simulink model "Charging_After_Balancing_16S1P"  (R2024b)
settings: Solver=VariableStepAuto  StartTime=0.0  StopTime=2500  RelTol=1e-3
undefined symbols (not defined in the file): Ion, Lithium
libraries: spsCurrentMeasurementLib x18, spsSeriesRLCBranchLib x17, spsVoltageMeasurementLib x17, spsBatteryLib x16, spsMosfetLib x16, spsIdealSwitchLib x2, spsDCVoltageSourceLib x1, spspowerguiLib x1
settings Model: SimulationMode=accelerator  Creator=HP
settings RTWCC: GPUComputeCapability=3.5

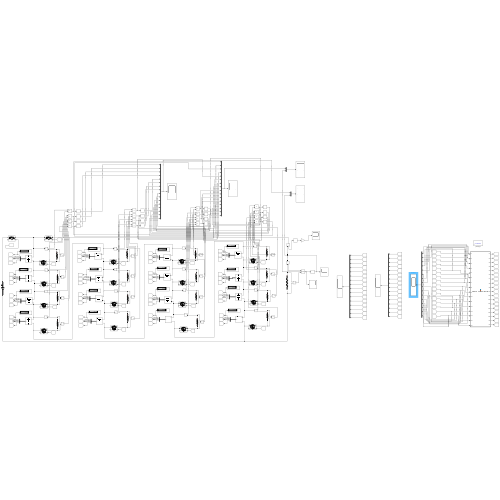
[thumbnail: Simulink's stored preview of the top-level diagram]
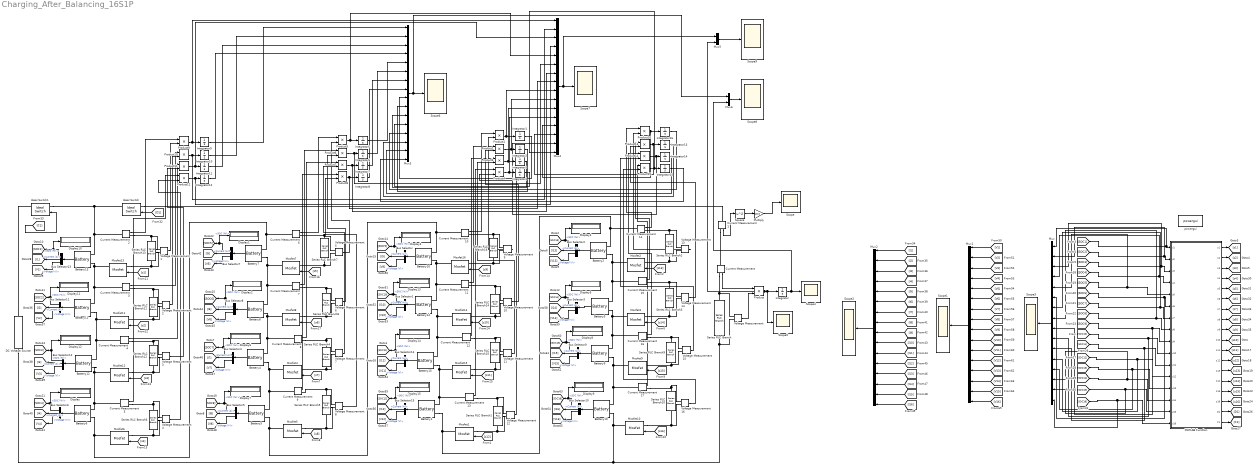
== system Charging_After_Balancing_16S1P ==
  Battery1 : spsBatteryLib/Battery  BatType=Lithium-Ion  NomV=3.3  NomQ=2.6  SOC=59  Batt_Tr=30  PresetModel=on  MaxQ=2.6  MinV=2.475  FullV=3.8412  Dis_rate=1.1304  R=0.012692  Normal_OP=2.3513  expZone="[3.5653     0.12774]"
  Battery10 : spsBatteryLib/Battery  BatType=Lithium-Ion  NomV=3.3  NomQ=2.6  SOC=55  Batt_Tr=30  PresetModel=on  MaxQ=2.6  MinV=2.475  FullV=3.8412  Dis_rate=1.1304  R=0.012692  Normal_OP=2.3513  expZone="[3.5653     0.12774]"
  Battery11 : spsBatteryLib/Battery  BatType=Lithium-Ion  NomV=3.3  NomQ=2.6  SOC=69  Batt_Tr=30  PresetModel=on  MaxQ=2.6  MinV=2.475  FullV=3.8412  Dis_rate=1.1304  R=0.012692  Normal_OP=2.3513  expZone="[3.5653     0.12774]"
  Battery12 : spsBatteryLib/Battery  BatType=Lithium-Ion  NomV=3.3  NomQ=2.6  SOC=68  Batt_Tr=30  PresetModel=on  MaxQ=2.6  MinV=2.475  FullV=3.8412  Dis_rate=1.1304  R=0.012692  Normal_OP=2.3513  expZone="[3.5653     0.12774]"
  Battery13 : spsBatteryLib/Battery  BatType=Lithium-Ion  NomV=3.3  NomQ=2.6  SOC=70  Batt_Tr=30  PresetModel=on  MaxQ=2.6  MinV=2.475  FullV=3.8412  Dis_rate=1.1304  R=0.012692  Normal_OP=2.3513  expZone="[3.5653     0.12774]"
  Battery14 : spsBatteryLib/Battery  BatType=Lithium-Ion  NomV=3.3  NomQ=2.6  SOC=61  Batt_Tr=30  PresetModel=on  MaxQ=2.6  MinV=2.475  FullV=3.8412  Dis_rate=1.1304  R=0.012692  Normal_OP=2.3513  expZone="[3.5653     0.12774]"
  Battery15 : spsBatteryLib/Battery  BatType=Lithium-Ion  NomV=3.3  NomQ=2.6  SOC=60  Batt_Tr=30  PresetModel=on  MaxQ=2.6  MinV=2.475  FullV=3.8412  Dis_rate=1.1304  R=0.012692  Normal_OP=2.3513  expZone="[3.5653     0.12774]"
  Battery16 : spsBatteryLib/Battery  BatType=Lithium-Ion  NomV=3.3  NomQ=2.6  SOC=62  Batt_Tr=30  PresetModel=on  MaxQ=2.6  MinV=2.475  FullV=3.8412  Dis_rate=1.1304  R=0.012692  Normal_OP=2.3513  expZone="[3.5653     0.12774]"
  Battery2 : spsBatteryLib/Battery  BatType=Lithium-Ion  NomV=3.3  NomQ=2.6  SOC=58  Batt_Tr=30  PresetModel=on  MaxQ=2.6  MinV=2.475  FullV=3.8412  Dis_rate=1.1304  R=0.012692  Normal_OP=2.3513  expZone="[3.5653     0.12774]"
  Battery3 : spsBatteryLib/Battery  BatType=Lithium-Ion  NomV=3.3  NomQ=2.6  SOC=57  Batt_Tr=30  PresetModel=on  MaxQ=2.6  MinV=2.475  FullV=3.8412  Dis_rate=1.1304  R=0.012692  Normal_OP=2.3513  expZone="[3.5653     0.12774]"
  Battery4 : spsBatteryLib/Battery  BatType=Lithium-Ion  NomV=3.3  NomQ=2.6  SOC=64  Batt_Tr=30  PresetModel=on  MaxQ=2.6  MinV=2.475  FullV=3.8412  Dis_rate=1.1304  R=0.012692  Normal_OP=2.3513  expZone="[3.5653     0.12774]"
  Battery5 : spsBatteryLib/Battery  BatType=Lithium-Ion  NomV=3.3  NomQ=2.6  SOC=63  Batt_Tr=30  PresetModel=on  MaxQ=2.6  MinV=2.475  FullV=3.8412  Dis_rate=1.1304  R=0.012692  Normal_OP=2.3513  expZone="[3.5653     0.12774]"
  Battery6 : spsBatteryLib/Battery  BatType=Lithium-Ion  NomV=3.3  NomQ=2.6  SOC=67  Batt_Tr=30  PresetModel=on  MaxQ=2.6  MinV=2.475  FullV=3.8412  Dis_rate=1.1304  R=0.012692  Normal_OP=2.3513  expZone="[3.5653     0.12774]"
  Battery7 : spsBatteryLib/Battery  BatType=Lithium-Ion  NomV=3.3  NomQ=2.6  SOC=66  Batt_Tr=30  PresetModel=on  MaxQ=2.6  MinV=2.475  FullV=3.8412  Dis_rate=1.1304  R=0.012692  Normal_OP=2.3513  expZone="[3.5653     0.12774]"
  Battery8 : spsBatteryLib/Battery  BatType=Lithium-Ion  NomV=3.3  NomQ=2.6  SOC=65  Batt_Tr=30  PresetModel=on  MaxQ=2.6  MinV=2.475  FullV=3.8412  Dis_rate=1.1304  R=0.012692  Normal_OP=2.3513  expZone="[3.5653     0.12774]"
  Battery9 : spsBatteryLib/Battery  BatType=Lithium-Ion  NomV=3.3  NomQ=2.6  SOC=56  Batt_Tr=30  PresetModel=on  MaxQ=2.6  MinV=2.475  FullV=3.8412  Dis_rate=1.1304  R=0.012692  Normal_OP=2.3513  expZone="[3.5653     0.12774]"
  Bus Selector{,1..15} (16 alike) : BusSelector  OutputSignals=SOC (%),Current (A),Voltage (V)
  Current Measurement{,1..17} (18 alike) : spsCurrentMeasurementLib/Current Measurement  PhasorSimulation=off  OutputType=Complex  PSBequivalent=0
  DC Voltage Source : spsDCVoltageSourceLib/DC Voltage Source  Amplitude=60  Measurements=None
  Display{,1..15} (16 alike) : Display
  Ideal Switch : spsIdealSwitchLib/Ideal Switch  Ron=0.001  Lon=0  IC=0  Rs=1e5  Cs=inf  Measurements=on
  Ideal Switch1 : spsIdealSwitchLib/Ideal Switch  Ron=0.001  Lon=0  IC=0  Rs=1e5  Cs=inf  Measurements=on
  Integrator{,1..16} (17 alike) : Integrator
  MATLAB Function : MATLAB Function  TreatAsAtomicUnit=on
  Mosfet{1..16} (16 alike) : spsMosfetLib/Mosfet  Ron=0.1  Lon=0  Rd=0.01  Vfd=0  IC=0  Rs=1e5  Cs=inf  Measurements=on
  Multiply : Gain  Gain=20.3
  Mux{,1..4} (5 alike) : Mux  Inputs=16
  Mux5 : Mux  Inputs=2
  Mux6 : Mux  Inputs=2
  Product{,1..16} (17 alike) : Product
  Scope{,1..9} (10 alike) : Scope
  Series RLC Branch : spsSeriesRLCBranchLib/Series RLC Branch  LConnTagsString=__new0  RConnTagsString=__new0  BranchType=R  Resistance=20.3  Inductance=1e-3  SetiL0=off  InitialCurrent=0  Capacitance=1e-6  Setx0=off  InitialVoltage=0  Measurements=None
  Series RLC Branch{1..16} (16 alike) : spsSeriesRLCBranchLib/Series RLC Branch  LConnTagsString=__new0  RConnTagsString=__new0  BranchType=R  Resistance=1.3  Inductance=1e-3  SetiL0=off  InitialCurrent=0  Capacitance=1e-6  Setx0=off  InitialVoltage=0  Measurements=None
  Square : Math  Operator=square
  Voltage Measurement{,1..16} (17 alike) : spsVoltageMeasurementLib/Voltage Measurement  PhasorSimulation=off  OutputType=Complex  PSBequivalent=0
  powergui : spspowerguiLib/powergui  Priority=1  SimulationMode=Continuous  SampleTime=50e-6  frequency=60  Iterations=50  frequencyindice=0  Pbase=100e6  ErrMax=1e-4  UnitsV=kV  UnitsW=MW  buscounter=0  FunctionMessages=off  echomessages=off  EnableUseOfTLC=off  CurrentSourceSwitches=off  DisableSnubberDevices=off  DisableRonSwitches=off  DisableVfSwitches=off  DisplayEquations=off  AutomaticDiscreteSolvers=off  SolverType=Tustin/Backward Euler (TBE)  Interpol=off  ExternalGateDelay=off  methode=off  Ts=100  x0status=blocks  SPID=on  SwTol=0  HookPort=off  NonlinearTolerance=1e-4  nMaxIteration=100  ContinueOnMaxIteration=off  RestoreLinks=warning  ResistiveCurrentMeasurement=off  Frange=[0:2:500]  Ylog=off  Xlog=on  ShowGrid=off  save=off  variable=ZData  structure=0  ZoomFFT=off  StartTime=0.0  cycles=1  DisplayStyle=1  fundamental=60  FreqAxis=off  MaxFrequency=1000  frequencyindicesteady=1  RmsSteady=1  display=off
  wires:
  MATLAB Function/1(s1) -> [s1]
  MATLAB Function/2(s2) -> [s2]
  MATLAB Function/3(s3) -> [s3]
  Battery6/1 -> Bus Selector6/1
  Battery7/1 -> Bus Selector7/1
  Battery8/1 -> Bus Selector8/1
  MATLAB Function/4(s4) -> [s4]
  MATLAB Function/5(s5) -> [s5]
  MATLAB Function/6(s6) -> [s6]
  MATLAB Function/7(s7) -> [s7]
  MATLAB Function/8(s8) -> [s8]
  MATLAB Function/9(s9) -> [s9]
  Bus Selector6/1 -> Display/1, [SOC4]  "<SOC (%)>"
  [s4] -> Mosfet6/1
  [s5] -> Mosfet7/1
  [s6] -> Mosfet8/1
  [s14] -> Mosfet3/1
  [s13] -> Mosfet2/1
  [s12] -> Mosfet1/1
  [s8] -> Mosfet5/1
  [s7] -> Mosfet4/1
  Battery5/1 -> Bus Selector5/1
  Battery4/1 -> Bus Selector4/1
  [s15] -> Mosfet9/1
  [s16] -> Mosfet10/1
  MATLAB Function/10(s10) -> [s10]
  Battery11/1 -> Bus Selector11/1
  Battery12/1 -> Bus Selector12/1
  Bus Selector11/1 -> Display11/1, [SOC2]  "<SOC (%)>"
  Bus Selector12/1 -> Display12/1, [SOC3]  "<SOC (%)>"
  [s2] -> Mosfet11/1
  [s3] -> Mosfet12/1
  [s1] -> Mosfet13/1
  Bus Selector13/1 -> Display10/1, [SOC1]  "<SOC (%)>"
  Battery13/1 -> Bus Selector13/1
  [s9] -> Mosfet16/1
  [s11] -> Mosfet15/1
  [s10] -> Mosfet14/1
  MATLAB Function/11(s11) -> [s11]
  MATLAB Function/12(s12) -> [s12]
  MATLAB Function/13(s13) -> [s13]
  MATLAB Function/14(s14) -> [s14]
  MATLAB Function/15(s15) -> [s15]
  MATLAB Function/16(s16) -> [s16]
  [SOC16] -> Mux/16, MATLAB Function/16(u16)
  [SOC15] -> MATLAB Function/15(u15), Mux/15
  [SOC14] -> Mux/14, MATLAB Function/14(u14)
  [SOC13] -> Mux/13, MATLAB Function/13(u13)
  [SOC12] -> Mux/12, MATLAB Function/12(u12)
  [SOC11] -> Mux/11, MATLAB Function/11(u11)
  [SOC10] -> Mux/10, MATLAB Function/10(u10)
  [SOC9] -> Mux/9, MATLAB Function/9(u9)
  [SOC8] -> Mux/8, MATLAB Function/8(u8)
  [SOC7] -> Mux/7, MATLAB Function/7(u7)
  [SOC6] -> Mux/6, MATLAB Function/6(u6)
  [SOC5] -> MATLAB Function/5(u5), Mux/5
  [SOC4] -> Mux/4, MATLAB Function/4(u4)
  [SOC3] -> Mux/3, MATLAB Function/3(u3)
  [SOC2] -> Mux/2, MATLAB Function/2(u2)
  [SOC1] -> Mux/1, MATLAB Function/1(u1)
  [D1] -> Ideal Switch/1
  MATLAB Function/17(D1) -> [D1]
  [C1] -> Ideal Switch1/1
  MATLAB Function/18(C1) -> [C1]
  Bus Selector11/2 -> [I2]  "<Current (A)>"
  Bus Selector11/3 -> [V2]  "<Voltage (V)>"
  Bus Selector12/2 -> [I3]  "<Current (A)>"
  Bus Selector12/3 -> [V3]  "<Voltage (V)>"
  Bus Selector6/2 -> [I4]  "<Current (A)>"
  Bus Selector6/3 -> [V4]  "<Voltage (V)>"
  Bus Selector13/2 -> [I1]  "<Current (A)>"
  Bus Selector13/3 -> [V1]  "<Voltage (V)>"
  Bus Selector5/1 -> Display7/1, [SOC8]  "<SOC (%)>"
  Bus Selector5/2 -> [I8]  "<Current (A)>"
  Bus Selector5/3 -> [V8]  "<Voltage (V)>"
  Bus Selector4/2 -> [I7]  "<Current (A)>"
  Bus Selector4/1 -> Display6/1, [SOC7]  "<SOC (%)>"
  Bus Selector4/3 -> [V7]  "<Voltage (V)>"
  Bus Selector8/1 -> Display2/1, [SOC6]  "<SOC (%)>"
  Battery16/1 -> Bus Selector/1
  Bus Selector1/2 -> [I10]  "<Current (A)>"
  Bus Selector1/1 -> Display13/1, [SOC10]  "<SOC (%)>"
  Bus Selector1/3 -> [V10]  "<Voltage (V)>"
  Bus Selector/2 -> [I9]  "<Current (A)>"
  Bus Selector/1 -> Display3/1, [SOC9]  "<SOC (%)>"
  Bus Selector/3 -> [V9]  "<Voltage (V)>"
  Bus Selector14/3 -> [V11]  "<Voltage (V)>"
  Bus Selector14/1 -> Display14/1, [SOC11]  "<SOC (%)>"
  Bus Selector14/2 -> [I11]  "<Current (A)>"
  Bus Selector15/2 -> [I12]  "<Current (A)>"
  Bus Selector15/1 -> Display15/1, [SOC12]  "<SOC (%)>"
  Bus Selector15/3 -> [V12]  "<Voltage (V)>"
  Battery15/1 -> Bus Selector14/1
  Battery1/1 -> Bus Selector15/1
  Bus Selector2/3 -> [V13]  "<Voltage (V)>"
  Bus Selector2/1 -> [SOC13], Display4/1  "<SOC (%)>"
  Bus Selector2/2 -> [I13]  "<Current (A)>"
  Bus Selector3/2 -> [I14]  "<Current (A)>"
  Bus Selector3/1 -> Display5/1, [SOC14]  "<SOC (%)>"
  Bus Selector3/3 -> [V14]  "<Voltage (V)>"
  Bus Selector9/3 -> [V15]  "<Voltage (V)>"
  Bus Selector9/1 -> [SOC15], Display8/1  "<SOC (%)>"
  Bus Selector9/2 -> [I15]  "<Current (A)>"
  Bus Selector10/2 -> [I16]  "<Current (A)>"
  Bus Selector10/1 -> Display9/1, [SOC16]  "<SOC (%)>"
  Bus Selector10/3 -> [V16]  "<Voltage (V)>"
  Battery14/1 -> Bus Selector1/1
  Battery2/1 -> Bus Selector2/1
  Battery3/1 -> Bus Selector3/1
  Battery9/1 -> Bus Selector9/1
  Battery10/1 -> Bus Selector10/1
  Bus Selector7/1 -> Display1/1, [SOC5]  "<SOC (%)>"
  Bus Selector7/2 -> [I5]  "<Current (A)>"
  Bus Selector7/3 -> [V5]  "<Voltage (V)>"
  [V1] -> Mux1/1
  [V2] -> Mux1/2
  [V3] -> Mux1/3
  [V4] -> Mux1/4
  [V5] -> Mux1/5
  [V6] -> Mux1/6
  [V7] -> Mux1/7
  [V8] -> Mux1/8
  [V9] -> Mux1/9
  [V10] -> Mux1/10
  [V11] -> Mux1/11
  [V12] -> Mux1/12
  [V13] -> Mux1/13
  [V14] -> Mux1/14
  [I1] -> Mux2/1
  [I2] -> Mux2/2
  [I3] -> Mux2/3
  [I4] -> Mux2/4
  [I5] -> Mux2/5
  [I6] -> Mux2/6
  [I7] -> Mux2/7
  [I8] -> Mux2/8
  [I9] -> Mux2/9
  [I10] -> Mux2/10
  [I11] -> Mux2/11
  [I12] -> Mux2/12
  [I13] -> Mux2/13
  [I14] -> Mux2/14
  [I15] -> Mux2/15
  [I16] -> Mux2/16
  [V15] -> Mux1/15
  [V16] -> Mux1/16
  Mux2/1 -> Scope2/1
  Mux1/1 -> Scope1/1
  Mux/1 -> Scope3/1
  Bus Selector8/2 -> [I6]  "<Current (A)>"
  Bus Selector8/3 -> [V6]  "<Voltage (V)>"
  Current Measurement1/1 -> Square/1
  Square/1 -> Multiply/1
  Multiply/1 -> Scope/1
  Current Measurement/1 -> Product/1
  Voltage Measurement/1 -> Product/2
  Product/1 -> Scope5/1, Integrator/1, Mux5/2
  Integrator/1 -> Mux6/2, Scope4/1
  Product1/1 -> Mux4/9, Integrator1/1
  Product2/1 -> Mux4/10, Integrator2/1
  Product3/1 -> Mux4/11, Integrator3/1
  Product4/1 -> Integrator4/1, Mux4/12
  Product8/1 -> Mux4/8, Integrator8/1
  Product7/1 -> Mux4/7, Integrator7/1
  Product6/1 -> Mux4/6, Integrator6/1
  Product5/1 -> Mux4/5, Integrator5/1
  Product9/1 -> Mux4/1, Integrator9/1
  Product10/1 -> Mux4/2, Integrator10/1
  Product11/1 -> Mux4/3, Integrator11/1
  Product12/1 -> Mux4/4, Integrator12/1
  Product15/1 -> Mux4/16, Integrator15/1
  Product14/1 -> Mux4/15, Integrator14/1
  Product13/1 -> Mux4/14, Integrator13/1
  Product16/1 -> Mux4/13, Integrator16/1
  Current Measurement2/1 -> Product9/1
  Voltage Measurement1/1 -> Product9/2
  Current Measurement3/1 -> Product10/1
  Voltage Measurement2/1 -> Product10/2
  Current Measurement4/1 -> Product11/1
  Voltage Measurement3/1 -> Product11/2
  Current Measurement5/1 -> Product12/1
  Voltage Measurement4/1 -> Product12/2
  Current Measurement6/1 -> Product5/1
  Voltage Measurement5/1 -> Product5/2
  Current Measurement7/1 -> Product6/1
  Voltage Measurement6/1 -> Product6/2
  Current Measurement8/1 -> Product7/1
  Voltage Measurement7/1 -> Product7/2
  Current Measurement9/1 -> Product8/1
  Voltage Measurement8/1 -> Product8/2
  Current Measurement10/1 -> Product1/1
  Voltage Measurement9/1 -> Product1/2
  Current Measurement11/1 -> Product2/1
  Voltage Measurement10/1 -> Product2/2
  Current Measurement12/1 -> Product3/1
  Voltage Measurement11/1 -> Product3/2
  Current Measurement13/1 -> Product4/1
  Voltage Measurement12/1 -> Product4/2
  Current Measurement14/1 -> Product16/1
  Voltage Measurement13/1 -> Product16/2
  Current Measurement15/1 -> Product13/1
  Voltage Measurement14/1 -> Product13/2
  Current Measurement16/1 -> Product14/1
  Voltage Measurement15/1 -> Product14/2
  Current Measurement17/1 -> Product15/1
  Voltage Measurement16/1 -> Product15/2
  Integrator9/1 -> Mux3/1
  Integrator10/1 -> Mux3/2
  Integrator11/1 -> Mux3/3
  Integrator12/1 -> Mux3/4
  Integrator5/1 -> Mux3/5
  Integrator6/1 -> Mux3/6
  Integrator7/1 -> Mux3/7
  Integrator8/1 -> Mux3/8
  Integrator1/1 -> Mux3/9
  Integrator2/1 -> Mux3/10
  Integrator3/1 -> Mux3/11
  Integrator4/1 -> Mux3/12
  Integrator16/1 -> Mux3/13
  Integrator13/1 -> Mux3/14
  Integrator14/1 -> Mux3/15
  Integrator15/1 -> Mux3/16
  Mux3/1 -> Mux6/1, Scope6/1
  Mux4/1 -> Mux5/1, Scope7/1
  Mux5/1 -> Scope9/1
  Mux6/1 -> Scope8/1
  connections:
  Mosfet6/LConn1 -- Voltage Measurement4/LConn2 -- Series RLC Branch6/RConn1
  Series RLC Branch7/RConn1 -- Voltage Measurement5/LConn2 -- Mosfet7/LConn1
  Mosfet8/LConn1 -- Voltage Measurement6/LConn2 -- Series RLC Branch8/RConn1
  Series RLC Branch3/LConn1 -- Current Measurement15/RConn1 -- Voltage Measurement14/LConn1
  Series RLC Branch2/RConn1 -- Mosfet2/LConn1 -- Voltage Measurement13/LConn2
  Mosfet1/LConn1 -- Voltage Measurement12/LConn2 -- Series RLC Branch1/RConn1
  Mosfet3/LConn1 -- Voltage Measurement14/LConn2 -- Series RLC Branch3/RConn1
  Voltage Measurement8/LConn1 -- Series RLC Branch5/LConn1 -- Current Measurement9/RConn1
  Mosfet5/LConn1 -- Voltage Measurement8/LConn2 -- Series RLC Branch5/RConn1
  Series RLC Branch4/RConn1 -- Mosfet4/LConn1 -- Voltage Measurement7/LConn2
  Battery9/LConn2 -- Mosfet9/RConn1 -- Current Measurement17/LConn1 -- Battery10/LConn1
  Series RLC Branch9/RConn1 -- Voltage Measurement15/LConn2 -- Mosfet9/LConn1
  Mosfet10/LConn1 -- Series RLC Branch10/RConn1 -- Voltage Measurement16/LConn2
  Voltage Measurement7/LConn1 -- Current Measurement8/RConn1 -- Series RLC Branch4/LConn1
  Series RLC Branch9/LConn1 -- Current Measurement16/RConn1 -- Voltage Measurement15/LConn1
  Battery11/LConn2 -- Mosfet11/RConn1 -- Current Measurement4/LConn1 -- Battery12/LConn1
  Voltage Measurement2/LConn1 -- Current Measurement3/RConn1 -- Series RLC Branch11/LConn1
  Series RLC Branch11/RConn1 -- Mosfet11/LConn1 -- Voltage Measurement2/LConn2
  Mosfet12/LConn1 -- Voltage Measurement3/LConn2 -- Series RLC Branch12/RConn1
  Mosfet13/LConn1 -- Voltage Measurement1/LConn2 -- Series RLC Branch13/RConn1
  Voltage Measurement11/LConn1 -- Current Measurement12/RConn1 -- Series RLC Branch15/LConn1
  Series RLC Branch14/LConn1 -- Current Measurement11/RConn1 -- Voltage Measurement10/LConn1
  Mosfet16/LConn1 -- Voltage Measurement9/LConn2 -- Series RLC Branch16/RConn1
  Series RLC Branch14/RConn1 -- Mosfet14/LConn1 -- Voltage Measurement10/LConn2
  Mosfet15/LConn1 -- Voltage Measurement11/LConn2 -- Series RLC Branch15/RConn1
  Battery12/LConn2 -- Mosfet12/RConn1 -- Current Measurement5/LConn1 -- Battery6/LConn1
  Series RLC Branch1/LConn1 -- Current Measurement13/RConn1 -- Voltage Measurement12/LConn1
  Battery7/LConn2 -- Mosfet7/RConn1 -- Current Measurement7/LConn1 -- Battery8/LConn1
  Series RLC Branch7/LConn1 -- Voltage Measurement5/LConn1 -- Current Measurement6/RConn1
  Battery5/LConn2 -- Current Measurement10/LConn1 -- Battery16/LConn1 -- Mosfet5/RConn1
  Battery1/LConn2 -- Mosfet1/RConn1 -- Current Measurement14/LConn1 -- Battery2/LConn1
  Ideal Switch1/LConn1 -- Ideal Switch/RConn1 -- Current Measurement2/LConn1 -- Battery13/LConn1
  Battery10/LConn2 -- Mosfet10/RConn1 -- DC Voltage Source/LConn1 -- Series RLC Branch/RConn1 -- Voltage Measurement/LConn2
  Current Measurement/RConn1 -- Voltage Measurement/LConn1 -- Series RLC Branch/LConn1
  DC Voltage Source/RConn1 -- Ideal Switch1/RConn1
  Ideal Switch/LConn1 -- Current Measurement1/LConn1
  Current Measurement1/RConn1 -- Current Measurement/LConn1
  Voltage Measurement1/LConn1 -- Current Measurement2/RConn1 -- Series RLC Branch13/LConn1
  Battery13/LConn2 -- Mosfet13/RConn1 -- Current Measurement3/LConn1 -- Battery11/LConn1
  Voltage Measurement3/LConn1 -- Current Measurement4/RConn1 -- Series RLC Branch12/LConn1
  Voltage Measurement4/LConn1 -- Current Measurement5/RConn1 -- Series RLC Branch6/LConn1
  Mosfet6/RConn1 -- Battery6/LConn2 -- Current Measurement6/LConn1 -- Battery7/LConn1
  Voltage Measurement6/LConn1 -- Current Measurement7/RConn1 -- Series RLC Branch8/LConn1
  Battery8/LConn2 -- Mosfet8/RConn1 -- Current Measurement8/LConn1 -- Battery4/LConn1
  Battery4/LConn2 -- Mosfet4/RConn1 -- Battery5/LConn1 -- Current Measurement9/LConn1
  Series RLC Branch16/LConn1 -- Current Measurement10/RConn1 -- Voltage Measurement9/LConn1
  Battery16/LConn2 -- Current Measurement11/LConn1 -- Battery14/LConn1 -- Mosfet16/RConn1
  Mosfet14/RConn1 -- Current Measurement12/LConn1 -- Battery15/LConn1 -- Battery14/LConn2
  Battery15/LConn2 -- Mosfet15/RConn1 -- Current Measurement13/LConn1 -- Battery1/LConn1
  Series RLC Branch2/LConn1 -- Voltage Measurement13/LConn1 -- Current Measurement14/RConn1
  Mosfet2/RConn1 -- Battery2/LConn2 -- Current Measurement15/LConn1 -- Battery3/LConn1
  Battery3/LConn2 -- Mosfet3/RConn1 -- Current Measurement16/LConn1 -- Battery9/LConn1
  Series RLC Branch10/LConn1 -- Voltage Measurement16/LConn1 -- Current Measurement17/RConn1

== matlab function Charging_After_Balancing_16S1P/MATLAB Function ==
  data: u1 input; s1 output; u2 input; u3 input; s2 output; s3 output; u4 input; u5 input; u6 input; u7 input; u8 input; u9 input; s4 output; s5 output; s6 output; s7 output; s8 output; s9 output; s10 output; u10 input; u11 input; u12 input; u13 input; u14 input; u15 input; u16 input; s11 output; s12 output; s13 output; s14 output; s15 output; s16 output; D1 output; C1 output
function [s1, s2, s3, s4, s5, s6, s7, s8, s9, s10, s11, s12, s13, s14, s15, s16, D1, C1] = passive_balancing_16S1P(u1,u2,u3,u4,u5,u6,u7,u8,u9,u10,u11,u12,u13,u14,u15,u16)

% Threshold limit for balancing (e.g., 0.2% SoC)
threshold = 0.2;

% Create array of all cell SoCs
soc = [u1,u2,u3,u4,u5,u6,u7,u8,u9,u10,u11,u12,u13,u14,u15,u16];

% Initialize switches (0 = OFF, 1 = ON)
s = zeros(1,16);  D1=0;

% Find minimum SoC
min_soc = min(soc);

% Balancing Phase: If any cell > (min_soc + threshold), turn ON its switch
for i = 1:16
    if soc(i) > (min_soc + threshold)
        s(i) = 1;  % Turn ON balancing switch
    else
        s(i) = 0;  % Switch OFF
    end
end

% Check if balancing is done (all differences within threshold)
if all((soc - min_soc) <= threshold)
    C1 = 1;  % Start discharging
else
    C1 = 0;  % Discharge OFF until balanced
end

% Assign outputs
s1 = s(1); s2 = s(2); s3 = s(3); s4 = s(4); s5 = s(5); s6 = s(6); s7 = s(7); s8 = s(8);
s9 = s(9); s10 = s(10); s11 = s(11); s12 = s(12); s13 = s(13); s14 = s(14); s15 = s(15); s16 = s(16);

end
